simulink model "main_direct"  (R2022b)
settings: Solver=ode45  StartTime=0.0  StopTime=5  RelTol=1e-3  EnableMultiTasking=on
InitFcn:
  | clear functions
  | initialize
values from neighbouring files (symbols this model uses):
  A_cc = [0 1 0 ... (first row only)    [initialize.m]
  A_esp = [-16.95,  -2.365 ... (first row only)    [initialize.m]
  A_sc = [3.957e-14  1  1.351e-14   1.193e-16 ... (first row only)    [initialize.m]
  A_ttc = [0,1;0,0]    [initialize.m]
  B_cc = [0; 0; 2.4767]    [initialize.m]
  B_esp = [8.478 ... (first row only)    [initialize.m]
  B_sc = [9.628e-15; 80; 20; -1120]    [initialize.m]
  B_ttc = [0;1]    [initialize.m]
  C_cc = [1 0 0]    [initialize.m]
  C_esp = [0,1]    [initialize.m]
  C_sc = [1 0 0 0]    [initialize.m]
  C_ttc = [1,0]    [initialize.m]
  D_cc = [0]    [initialize.m]
  D_esp = [0]    [initialize.m]
  D_sc = [0]    [initialize.m]
  D_ttc = [0]    [initialize.m]
undefined symbols (not defined in the file or in its folder): sharedmem
libraries: truetime x1
settings Model: Creator=anton  LastModifiedBy=sunan
settings SolverCC: AlgebraicLoopSolver=TrustRegion
settings DataIOCC: SaveFormat=Array  SignalLoggingSaveFormat=ModelDataLogs  ReturnWorkspaceOutputs=off
settings OptimizationCC: BlockReduction=off  BooleanDataType=off  ExpressionDepthLimit=2147483647  LifeSpan=inf
settings DebuggingCC: SaveWithParameterizedLinksMsg=none  UnderspecifiedInitializationDetection=Classic  MergeDetectMultiDrivingBlocksExec=none  SignalResolutionControl=TryResolveAllWithWarning  MultiTaskDSMMsg=warning  MultiTaskCondExecSysMsg=none  FcnCallInpInsideContextMsg=warning  UnconnectedInputMsg=warning  UnconnectedOutputMsg=warning  UnconnectedLineMsg=warning  StateNameClashWarn=warning  SFUnexpectedBacktrackingDiag=warning  SFNoUnconditionalDefaultTransitionDiag=warning  SFExecutionAtInitializationDiag=none  SFMachineParentedDataDiag=warning  ArithmeticOperatorsInVariantConditions=warning
settings HardwareCC: ProdBitPerPointer=32  ProdBitPerSizeT=32  ProdBitPerPtrDiffT=32  ProdLargestAtomicFloat=None  ProdIntDivRoundTo=Undefined  ProdEndianess=Unspecified  ProdWordSize=32  ProdHWDeviceType=32-bit Generic  TargetUnknown=on
settings ModelReferenceCC: EnableRefExpFcnMdlSchedulingChecks=on  PropagateSignalLabelsOutOfModel=off
settings SFSimCC: SimUseLocalCustomCode=off  CustomCodeUndefinedFunction=UseInterfaceOnly
settings RTWCC: RTWUseLocalCustomCode=off  DLArmComputeVersion=19.05
settings CodeAppCC: StateflowObjectComments=on
settings GRTTargetCC: TargetLangStandard=C89/C90 (ANSI)  CombineOutputUpdateFcns=off  GRTInterface=on
settings ConfigComp: CovMetricSettings=dw  CovSaveCumulativeToWorkspaceVar=on  CovSaveSingleToWorkspaceVar=on  CovExternalEMLEnable=off

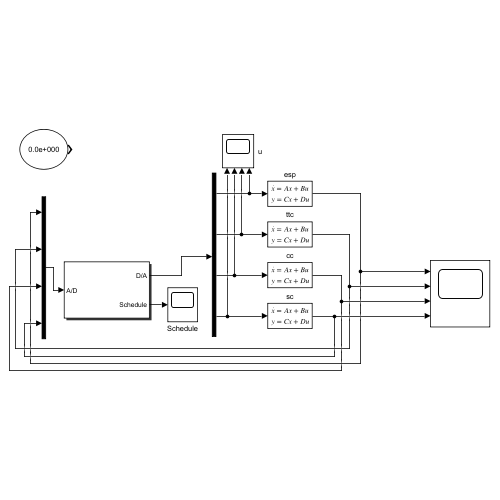
[thumbnail: Simulink's stored preview of the top-level diagram]
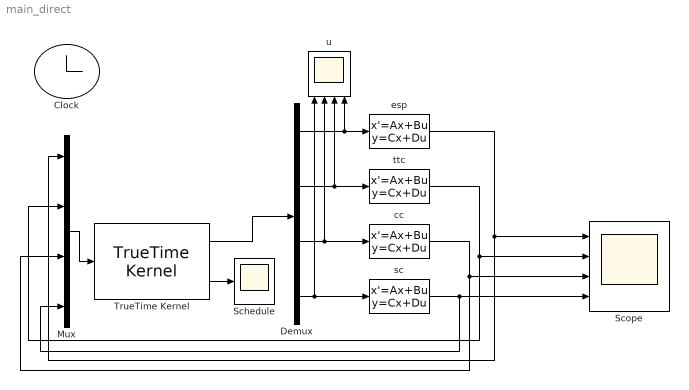
== system main_direct ==
  Clock : Clock
  Demux : Demux
      settings: DisplayOption=none
  Mux : Mux
  Schedule : Scope
  Scope : Scope  NumInputPorts=4
  TrueTime Kernel : truetime/TrueTime Kernel  sfun=control_sched_init  args=Systems  ninputsoutputs=[4 4]  ntriggers=0  trigtype=falling  nwnodenbr=[]  clockoffsetdrift=[0 0]  schedoutput=on  battery=off  poweroutput=off
  cc : StateSpace  A=A_cc  B=B_cc  C=C_cc  D=D_cc  InitialCondition=sharedmem.x0{3}
  esp : StateSpace  A=A_esp  B=B_esp  C=C_esp  D=D_esp  InitialCondition=sharedmem.x0{1}
  sc : StateSpace  A=A_sc  B=B_sc  C=C_sc  D=D_sc  InitialCondition=sharedmem.x0{4}
  ttc : StateSpace  A=A_ttc  B=B_ttc  C=C_ttc  D=D_ttc  InitialCondition=sharedmem.x0{2}
  u : Scope  NumInputPorts=4
  wires:
  esp/1 -> Scope/1, Mux/1
  sc/1 -> Scope/4, Mux/4
  Mux/1 -> TrueTime Kernel/1
  TrueTime Kernel/1 -> Demux/1
  cc/1 -> Scope/3, Mux/3
  ttc/1 -> Scope/2, Mux/2
  TrueTime Kernel/2 -> Schedule/1
  Demux/4 -> u/1, sc/1
  Demux/3 -> cc/1, u/2
  Demux/2 -> ttc/1, u/3
  Demux/1 -> esp/1, u/4
